simulink model "scuba_buoyancy_sim"  (R2026a)
settings: Solver=ode23t  StopTime=120  MaxStep=0.01
undefined symbols (not defined in the file): env_g, gas_T
libraries: scuba_lib x14, nesl_utility x6, fl_lib x3
settings Model: Creator=grouleau  LastModifiedBy=grouleau

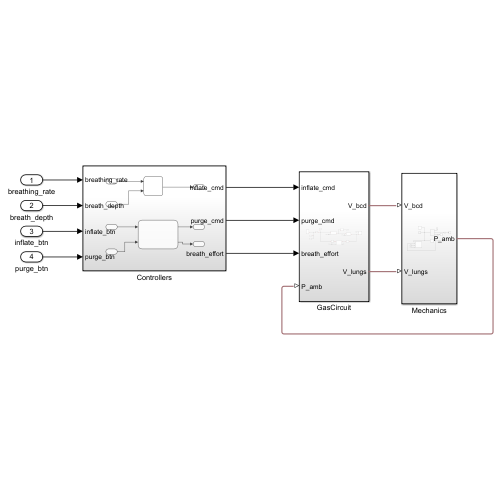
[thumbnail: Simulink's stored preview of the top-level diagram]
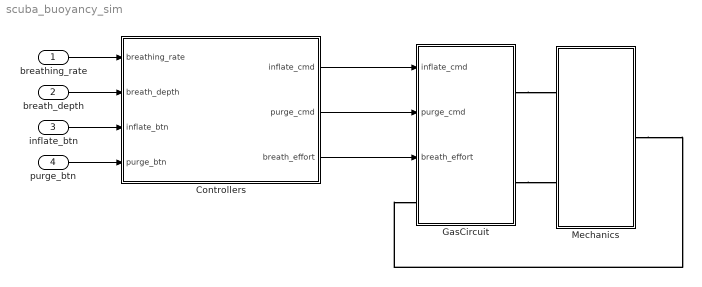
== system scuba_buoyancy_sim ==
  breathing_rate : Inport
  breath_depth : Inport  Port=2
  inflate_btn : Inport  Port=3
  purge_btn : Inport  Port=4
  Controllers : Subsystem
  GasCircuit : Subsystem
  Mechanics : Subsystem
  wires:
  breathing_rate/1 -> Controllers/1(breathing_rate)
  breath_depth/1 -> Controllers/2(breath_depth)
  inflate_btn/1 -> Controllers/3(inflate_btn)
  purge_btn/1 -> Controllers/4(purge_btn)
  Controllers/1(inflate_cmd) -> GasCircuit/1(inflate_cmd)
  Controllers/3(breath_effort) -> GasCircuit/3(breath_effort)
  Controllers/2(purge_cmd) -> GasCircuit/2(purge_cmd)
  connections:
  Mechanics/RConn1 -- GasCircuit/LConn1
  GasCircuit/RConn1 -- Mechanics/LConn1
  GasCircuit/RConn2 -- Mechanics/LConn2

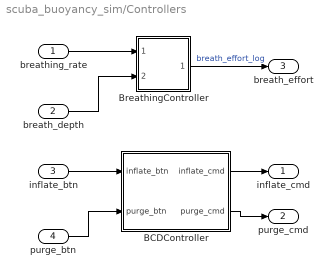
== system scuba_buoyancy_sim/Controllers ==
  breathing_rate : Inport
  breath_depth : Inport  Port=2
  inflate_btn : Inport  Port=3
  purge_btn : Inport  Port=4
  BCDController : Stateflow chart  TreatAsAtomicUnit=on
  BreathingController : Stateflow chart  TreatAsAtomicUnit=on
  inflate_cmd : Outport
  purge_cmd : Outport  Port=2
  breath_effort : Outport  Port=3
  wires:
  BCDController/2(purge_cmd) -> purge_cmd/1
  BreathingController/1(breath_effort) -> breath_effort/1  "breath_effort_log"
  BCDController/1(inflate_cmd) -> inflate_cmd/1
  breathing_rate/1 -> BreathingController/1(breathing_rate)
  breath_depth/1 -> BreathingController/2(breath_depth)
  inflate_btn/1 -> BCDController/1(inflate_btn)
  purge_btn/1 -> BCDController/2(purge_btn)

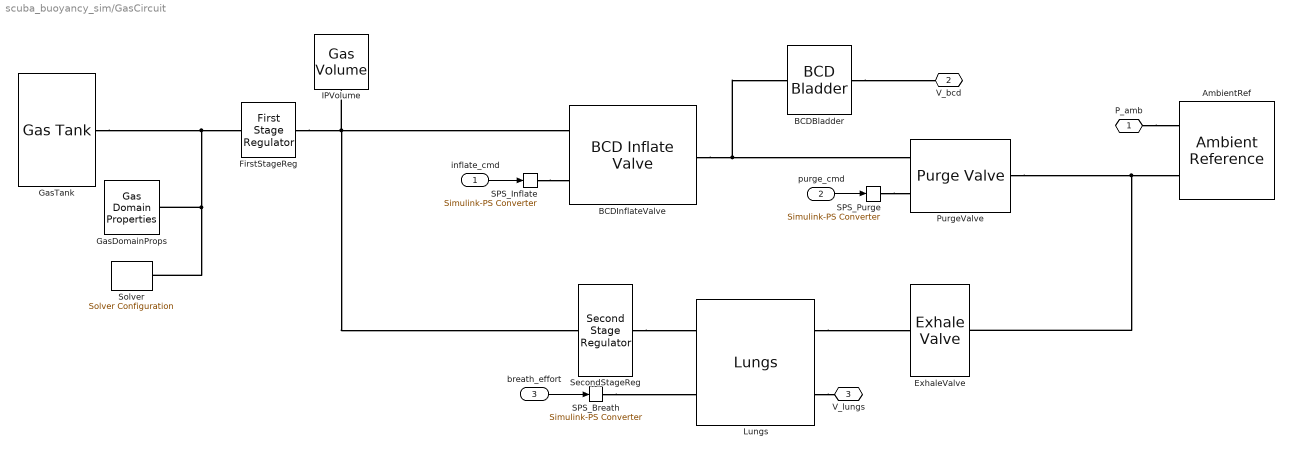
== system scuba_buoyancy_sim/GasCircuit ==
  inflate_cmd : Inport
  purge_cmd : Inport  Port=2
  breath_effort : Inport  Port=3
  AmbientRef : scuba_lib/gas/elements/Ambient Reference  n_dot_in_specify=off  n_dot_in_priority=None  n_dot_in=0 mol/s  n_dot_in_nominal_specify=off  n_dot_in_nominal_value=1  n_dot_in_nominal_unit=mol/s
  BCDBladder : scuba_lib/gas/elements/BCD Bladder  V_max=bcd_V_max m^3  n_init=bcd_n_init mol  K_wall=bcd_K_wall Pa/m^3  n_dot_in_specify=off  n_dot_in_priority=None  n_dot_in=0 mol/s  n_dot_in_nominal_specify=off  n_dot_in_nominal_value=1  n_dot_in_nominal_unit=mol/s
  BCDInflateValve : scuba_lib/gas/elements/BCD Inflate Valve  R_open=bcdinfl_R_open Pa*s/mol  n_dot_specify=off  n_dot_priority=None  n_dot=0 mol/s  n_dot_nominal_specify=off  n_dot_nominal_value=1  n_dot_nominal_unit=mol/s
  ExhaleValve : scuba_lib/gas/elements/Exhale Valve  P_crack=exhale_P_crack Pa  R_open=exhale_R_open Pa*s/mol  n_dot_specify=off  n_dot_priority=None  n_dot=0 mol/s  n_dot_nominal_specify=off  n_dot_nominal_value=1  n_dot_nominal_unit=mol/s
  FirstStageReg : scuba_lib/gas/elements/First Stage Regulator  IP_offset=reg1_IP_offset Pa  R_open=reg1_R_open Pa*s/mol  n_dot_specify=off  n_dot_priority=None  n_dot=0 mol/s  n_dot_nominal_specify=off  n_dot_nominal_value=1  n_dot_nominal_unit=mol/s
  GasDomainProps : scuba_lib/gas/elements/Gas Domain Properties  R_gas=gas_R J/(K*mol)  T=gas_T K  n_dot_thru_specify=off  n_dot_thru_priority=None  n_dot_thru=0 mol/s  n_dot_thru_nominal_specify=off  n_dot_thru_nominal_value=1  n_dot_thru_nominal_unit=mol/s
  GasTank : scuba_lib/gas/elements/Gas Tank  V_tank=tank_V m^3  n_init=tank_n_init mol  n_dot_out_specify=off  n_dot_out_priority=None  n_dot_out=0 mol/s  n_dot_out_nominal_specify=off  n_dot_out_nominal_value=1  n_dot_out_nominal_unit=mol/s
  IPVolume : scuba_lib/gas/elements/Gas Volume  V=ipvol_V m^3  n_init=ipvol_n_init mol  n_dot_in_specify=off  n_dot_in_priority=None  n_dot_in=0 mol/s  n_dot_in_nominal_specify=off  n_dot_in_nominal_value=1  n_dot_in_nominal_unit=mol/s
  Lungs : scuba_lib/gas/elements/Lungs  n_init=lungs_n_init mol  n_dot_in_specify=off  n_dot_in_priority=None  n_dot_in=0 mol/s  n_dot_in_nominal_specify=off  n_dot_in_nominal_value=1  n_dot_in_nominal_unit=mol/s  n_dot_out_specify=off  n_dot_out_priority=None  n_dot_out=0 mol/s  n_dot_out_nominal_specify=off  n_dot_out_nominal_value=1  n_dot_out_nominal_unit=mol/s
  PurgeValve : scuba_lib/gas/elements/Purge Valve  R_open=purge_R_open Pa*s/mol  n_dot_specify=off  n_dot_priority=None  n_dot=0 mol/s  n_dot_nominal_specify=off  n_dot_nominal_value=1  n_dot_nominal_unit=mol/s
  SPS_Breath : nesl_utility/Simulink-PS Converter  PhysicalDomain=network_engine_domain  SubClassName=ps_input  LeftPortType=input  RightPortType=output  PseudoPeriodic=off  Frequencies=[]  NoiseDistribution=none  NoiseParameters=[]  Unit=Pa  AffineConversion=off  FilteringAndDerivatives=provide  SimscapeFilterOrder=1  InputFilterTimeConstant=0.001  UdotUserProvided=0
  SPS_Inflate : nesl_utility/Simulink-PS Converter  PhysicalDomain=network_engine_domain  SubClassName=ps_input  LeftPortType=input  RightPortType=output  PseudoPeriodic=off  Frequencies=[]  NoiseDistribution=none  NoiseParameters=[]  Unit=1  AffineConversion=off  FilteringAndDerivatives=provide  SimscapeFilterOrder=1  InputFilterTimeConstant=0.001  UdotUserProvided=0
  SPS_Purge : nesl_utility/Simulink-PS Converter  PhysicalDomain=network_engine_domain  SubClassName=ps_input  LeftPortType=input  RightPortType=output  PseudoPeriodic=off  Frequencies=[]  NoiseDistribution=none  NoiseParameters=[]  Unit=1  AffineConversion=off  FilteringAndDerivatives=provide  SimscapeFilterOrder=1  InputFilterTimeConstant=0.001  UdotUserProvided=0
  SecondStageReg : scuba_lib/gas/elements/Second Stage Regulator  P_crack=reg2_P_crack Pa  R_open=reg2_R_open Pa*s/mol  n_dot_specify=off  n_dot_priority=None  n_dot=0 mol/s  n_dot_nominal_specify=off  n_dot_nominal_value=1  n_dot_nominal_unit=mol/s
  Solver : nesl_utility/Solver Configuration  PhysicalDomain=network_engine_domain  SubClassName=solver  LeftPortType=input  RightPortType=generic  Tones=[]  Harmonics=[]  SimulateNoise=off  Profile=off  UseLocalSampling=off  EnableSwitchedLinearOptims=on  FrequencyDomain=off  UseCCode=off  RelTol=0.001  AbsTol=0.001  MinStep=1e-09  ToWorkspace=off  RevertToSquareIcSolve=off  NumHomotopyIterations=100  PhasorMode=off  PhasorModeNumHarmonics=1  ConsistencySolver=NEWTON_XTOL_AFTER_FTOL  CanonicalOrdering=CANONICAL  OptimizeIntermediates=OPTIMIZED  IndexReductionMethod=DerivativeReplacement  DoDC=off  ResidualTolerance=1e-09  ConsistencyTolSource=GLOBAL  ConsistencyAbsTol=0.001  ConsistencyRelTol=0.001  ConsistencyTolFactor=0.001  UseLocalSolver=off  LocalSolverChoice=NE_BACKWARD_EULER_ADVANCER  ResolveIndetEquations=on  FunctionEvalNumThread=1  LocalSolverSampleTime=0.001  DoFixedCost=off  MaxNonlinIter=3  MaxModeIter=2  ComputeImpulses=off  ImpulseIterations=2  LinearAlgebra=auto  LinearAlgebraNumThread=0  EquationFormulation=NE_TIME_EF  DelaysMemoryBudget=1024  AutomaticFiltering=on  FilteringTimeConstant=0.001  PartitionStorageMethod=AS_NEEDED  PartitionMemoryBudget=1024  PartitionMethod=ROBUST  MultibodyUseLocalSolver=off  MultibodyLocalSolverChoice=ODE1  MultibodyLocalSolverSampleTime=0.001
  P_amb : PMIOPort  Side=Left
  V_bcd : PMIOPort  Port=2  Side=Right
  V_lungs : PMIOPort  Port=3  Side=Right
  wires:
  purge_cmd/1 -> SPS_Purge/1
  inflate_cmd/1 -> SPS_Inflate/1
  breath_effort/1 -> SPS_Breath/1
  connections:
  SPS_Purge/RConn1 -- PurgeValve/LConn2
  SPS_Inflate/RConn1 -- BCDInflateValve/LConn2
  GasTank/RConn1 -- Solver/RConn1 -- GasDomainProps/LConn1 -- FirstStageReg/LConn1
  P_amb/RConn1 -- AmbientRef/LConn2
  Lungs/RConn2 -- V_lungs/RConn1
  FirstStageReg/RConn1 -- IPVolume/LConn1 -- SecondStageReg/LConn1 -- BCDInflateValve/LConn1
  BCDBladder/RConn1 -- V_bcd/RConn1
  BCDInflateValve/RConn1 -- BCDBladder/LConn1 -- PurgeValve/LConn1
  SecondStageReg/RConn1 -- Lungs/LConn1
  SPS_Breath/RConn1 -- Lungs/LConn2
  PurgeValve/RConn1 -- ExhaleValve/RConn1 -- AmbientRef/LConn1
  Lungs/RConn1 -- ExhaleValve/LConn1

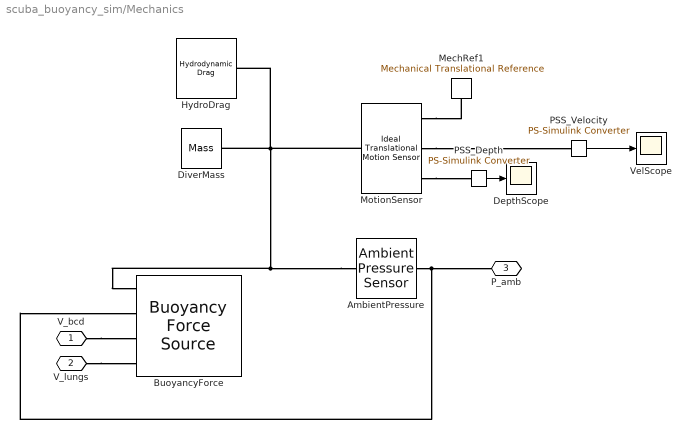
== system scuba_buoyancy_sim/Mechanics ==
  AmbientPressure : scuba_lib/Ambient Pressure Sensor  rho_water=env_rho_water kg/m^3  g=env_g m/s^2  P_atm=env_P_atm Pa  depth_init=ic_depth m  f_specify=off  f_priority=None  f=0 N  f_nominal_specify=off  f_nominal_value=1  f_nominal_unit=N
  BuoyancyForce : scuba_lib/Buoyancy Force Source  rho_water=env_rho_water kg/m^3  g=env_g m/s^2  P_atm=env_P_atm Pa  m_total=diver_m_total kg  V_body=diver_V_body m^3  V_gear=gear_V m^3  V_ws_surface=ws_V_surface m^3  compression_exp=ws_comp_exp  f_specify=off  f_priority=None  f=0 N  f_nominal_specify=off  f_nominal_value=1  f_nominal_unit=N
  DepthScope : Scope
  DiverMass : fl_lib/Mechanical/Translational Elements/Mass  mass=diver_mass_total kg  num_ports=foundation.enum.numPorts2.one  v_specify=on  v_priority=High  v=0 m/s  v_nominal_specify=off  v_nominal_value=1  v_nominal_unit=m/s  f_specify=off  f_priority=None  f=0 N  f_nominal_specify=off  f_nominal_value=1  f_nominal_unit=N
  HydroDrag : scuba_lib/Hydrodynamic Drag  rho_water=env_rho_water kg/m^3  Cd=drag_Cd  A_frontal=drag_A_frontal m^2  f_specify=off  f_priority=None  f=0 N  f_nominal_specify=off  f_nominal_value=1  f_nominal_unit=N
  MechRef1 : fl_lib/Mechanical/Translational Elements/Mechanical Translational Reference
  MotionSensor : fl_lib/Mechanical/Mechanical Sensors/Ideal Translational Motion Sensor  reference=foundation.enum.MeasurementReference.difference  acceleration_port=false  velocity_port=true  position_port=true  offset=0 m
  PSS_Depth : nesl_utility/PS-Simulink Converter  PhysicalDomain=network_engine_domain  SubClassName=ps_output  LeftPortType=input  RightPortType=output  PseudoPeriodic=off  Frequencies=[]  VectorFormat=inherit  Unit=m  AffineConversion=off
  PSS_Velocity : nesl_utility/PS-Simulink Converter  PhysicalDomain=network_engine_domain  SubClassName=ps_output  LeftPortType=input  RightPortType=output  PseudoPeriodic=off  Frequencies=[]  VectorFormat=inherit  Unit=m/s  AffineConversion=off
  VelScope : Scope
  V_bcd : PMIOPort  Side=Left
  V_lungs : PMIOPort  Port=2  Side=Left
  P_amb : PMIOPort  Port=3  Side=Right
  wires:
  PSS_Velocity/1 -> VelScope/1
  PSS_Depth/1 -> DepthScope/1
  connections:
  AmbientPressure/LConn1 -- BuoyancyForce/LConn1 -- HydroDrag/LConn1 -- DiverMass/LConn1 -- MotionSensor/LConn1
  V_bcd/RConn1 -- BuoyancyForce/LConn3
  AmbientPressure/RConn1 -- P_amb/RConn1 -- BuoyancyForce/LConn2
  MotionSensor/RConn1 -- MechRef1/LConn1
  MotionSensor/RConn3 -- PSS_Depth/LConn1
  MotionSensor/RConn2 -- PSS_Velocity/LConn1
  V_lungs/RConn1 -- BuoyancyForce/LConn4

== stateflow chart scuba_buoyancy_sim/Controllers/BCDController ==
  settings: updateMethod=DISCRETE  sampleTime=0.01
  state IDLE
    entry: inflate_cmd = 0; purge_cmd = 0;
  state PURGING
    entry: inflate_cmd = 0; purge_cmd = 1;
  state INFLATING
    entry: inflate_cmd = 1; purge_cmd = 0;
  (default) -> IDLE
  IDLE -> PURGING [order 2] : [purge_btn > 0.5 && inflate_btn < 0.5]
  PURGING -> IDLE [order 1] : [purge_btn < 0.5]
  IDLE -> INFLATING [order 1] : [inflate_btn > 0.5]
  INFLATING -> IDLE : [inflate_btn < 0.5]
  PURGING -> INFLATING [order 2] : [inflate_btn > 0.5]
  data: inflate_btn input; purge_btn input; inflate_cmd output; purge_cmd output

== stateflow chart scuba_buoyancy_sim/Controllers/BreathingController ==
  settings: updateMethod=DISCRETE  sampleTime=0.01
  state INHALE
    entry: t_phase = 0;
    during: T_cycle = 60/breathing_rate; T_inh = 0.40*T_cycle; breath_effort = -200*breath_depth*sin(pi*t_phase/T_inh); t_phase = t_phase + 0.01;
  state PAUSE_POST_INHALE
    entry: t_phase = 0;
    during: breath_effort = 0; t_phase = t_phase + 0.01;
  state EXHALE
    entry: t_phase = 0;
    during: T_cycle = 60/breathing_rate; T_exh = 0.35*T_cycle; breath_effort = 200*breath_depth*sin(pi*t_phase/T_exh); t_phase = t_phase + 0.01;
  state PAUSE_POST_EXHALE
    entry: t_phase = 0;
    during: breath_effort = 0; t_phase = t_phase + 0.01;
  (default) -> INHALE
  INHALE -> PAUSE_POST_INHALE : [t_phase >= 0.40*60/breathing_rate]
  PAUSE_POST_EXHALE -> INHALE : [t_phase >= 0.15*60/breathing_rate]
  PAUSE_POST_INHALE -> EXHALE : [t_phase >= 0.10*60/breathing_rate]
  EXHALE -> PAUSE_POST_EXHALE : [t_phase >= 0.35*60/breathing_rate]
  data: breathing_rate input; breath_depth input; breath_effort output; t_phase local =0; T_cycle local =4; T_inh local =1.6; T_exh local =1.4
